simulink model "sm_planetary_gear_testrig"  (R2026a)
settings: Solver=ode45  StopTime=30  MaxStep=0.01  AbsTol=1e-4  EnableMultiTasking=on
PreLoadFcn:
  | rad_planet = 0.26;
  | rad_sun = 0.78;
  | rad_ring = 2*rad_planet+rad_sun;
  | gear_thickness = 0.5;
  | link_thickness = 0.1;
  | rad_hole = 0.05;
InitFcn:
  | sun_xcdata=Extr_Data_Gear('external',rad_sun*2,45,rad_hole);
  | planet_xcdata=Extr_Data_Gear('external',rad_planet*2,15,rad_hole);
  | ring_xcdata=Extr_Data_Gear('internal',rad_ring*2,75,rad_ring*0.05);
undefined symbols (not defined in the file or in its folder): Local, sigbuilder_block, X, Y, Z
libraries: sm_lib x22, Multibody_Parts_Lib x15, nesl_utility x7, fl_lib x3
CloseFcn:
  | try,close(h1_sm_planetary_gear_testrig),end
  | clear h1_sm_planetary_gear_testrig
  | 
  | clear simlog_sm_planetary_gear_testrig
  | clear logsout_sm_planetary_gear_testrig
Description:
  | Planetary Gear Testrig
  | 
  | Copyright 2013-2026 The MathWorks, Inc.
settings Model: Creator=smiller  LastModifiedBy=smiller
settings DataIOCC: MaxDataPoints=20000  SignalLoggingName=logsout_sm_planetary_gear_testrig
settings DebuggingCC: UnderspecifiedInitializationDetection=Classic  PregeneratedLibrarySubsystemCodeDiagnostic=none
settings HardwareCC: ProdHWDeviceType=32-bit Generic
settings SimscapeCC: SimscapeNormalizeSystem=off  SimscapeNominalValues="[{\"value\":\"1\",\"unit\":\"A\"},{\"value\":\"1\",\"unit\":\"bar\"},{\"value\":\"1\",\"unit\":\"cm^2\"},{\"value\":\"1\",\"unit\":\"cm^3/s\"},{\"value\":\"1\",\"unit\":\"kJ/kg\"},{\"value\":\"1\",\"unit\":\"kW\"},{\"value\":\"1\",\"unit\":\"l\"},{\"value\":\"1\",\"unit\":\"N\"},{\"value\":\"1\",\"unit\":\"N*m\"},{\"value\":\"1\",\"unit\":\"V\"}]"  SimscapeLogSimulationStatistics=on  SimscapeLogName=simlog_sm_planetary_gear_testrig  SimscapeLogDataHistory=20000.0
settings ConfigurationSet: Description=SimMechanics 2G
settings ExplorerConfigSet: InternalSimMechanicsExplorerSettings="<ExplorerConfiguration><canonicalview>default</canonicalview><AnimationSetting><BasePlaybackSpeed>1.0</BasePlaybackSpeed><PlaybackSpeedFactor>4.0</PlaybackSpeedFactor></AnimationSetting><TilePanel><TileInfo><Tiles Columns=\"1\" Count=\"1\" Rows=\"1\"><Column Weight=\"1\"/><Row Weight=\"1\"/><Tile Height=\"1\" Width=\"1\" X=\"0\" Y=\"0\"/></Tiles></TileInfo><SceneInfo><SceneViewer><BGColor><R>1</R><G>1</G><B>1</B></BGColor><Camera><DoPerspective>off</DoPerspective><Position><X>1.99828155084314307</X><Y>1.0003722576482561</Y><Z>4.2039432286769749</Z></Position><Center><X>0.00967718522444371843</X><Y>-0.00673071493915866625</Y><Z>0.289800264927272178</Z></Center><Up><X>-0.134695748421889611</X><Y>0.973996605340227584</Y><Z>-0.182174828510363152</Z></Up><ViewLimDist>1</ViewLimDist><YLim>2.34587518109692095</YLim><XLim>2.44514384132151186</XLim></Camera></SceneViewer></SceneInfo></TilePanel><MechEditorPanel><Cameras/><GfxPanelCameraMap/><VideoCreator><PlaybackSpeedRatio>1.0</PlaybackSpeedRatio><FrameRate>30</FrameRate><VideoFormat>Motion JPEG AVI</VideoFormat><FrameSize>auto</FrameSize></VideoCreator></MechEditorPanel></ExplorerConfiguration>"

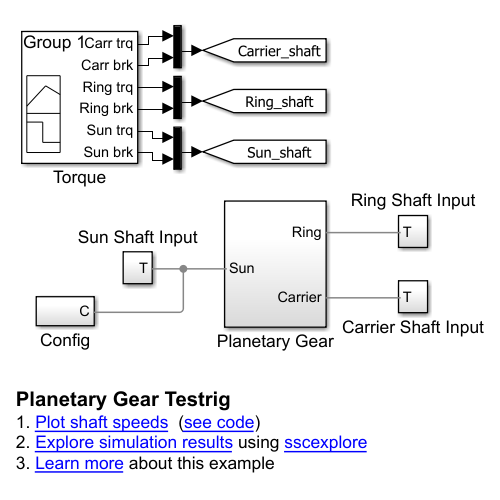
[thumbnail: Simulink's stored preview of the top-level diagram]
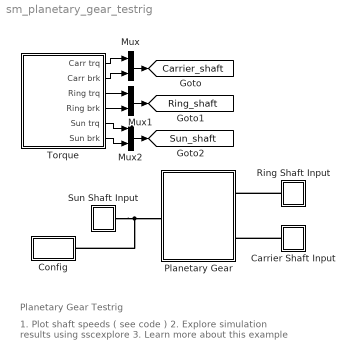
== system sm_planetary_gear_testrig ==
  note: Planetary Gear Testrig
  note: 1. Plot shaft speeds ( see code )
      | 2. Explore simulation results using sscexplore
      | 3. Learn more about this example
  Carrier Shaft Input : Subsystem
  Config : Subsystem
  Mux : Mux  Inputs=2
  Mux1 : Mux  Inputs=2
  Mux2 : Mux  Inputs=2
  Planetary Gear : Subsystem  Tag=PublishSubsystem
  Ring Shaft Input : Subsystem
  Sun Shaft Input : Subsystem  Tag=PublishSubsystem
  Torque : Subsystem  Tag=STV Subsys  LoadFcn=sigbuilder_block('load');  StartFcn=sigbuilder_block('start');  StopFcn=sigbuilder_block('stop');  ClipboardFcn=sigbuilder_block('clipboard');  mask(Sigbuilder block){tuvar=[0:10]}
      mask help: Simulink:masks:SigbuilderBlock_MD
      mask init:
      | if ~strcmp(get_param(bdroot(gcbh),'SimulationStatus'),'stopped') tuvar = sigbuilder_block('maskInit'); end
      settings: CopyFcn=sigbuilder_block('copy');  DeleteFcn=sigbuilder_block('delete');  ModelCloseFcn=sigbuilder_block('modelClose');  PreSaveFcn=sigbuilder_block('preSave');  PauseFcn=sigbuilder_block('pause');  ContinueFcn=sigbuilder_block('continue');  NameChangeFcn=sigbuilder_block('namechange');  OpenFcn=sigbuilder_block('open',[23.4 13.8 618.6 562.8 ]);  CloseFcn=sigbuilder_block('close');
      mask Display: plot(0, 0, 100, 100,[2, 2, 32, 32, 2], [68, 8, 8, 68, 68],[32, 2], [38, 38], [32, 19, 2],[53, 60, 44], [32, 17, 17, 2],[16, 16, 31, 31]);txt = getActiveGroup(gcbh);text(2, 100, txt,'verticalAlignment', 'top');
  tag scope: Carrier_shaft=global, Ring_shaft=global, Sun_shaft=global
  wires:
  Torque/1(Carr trq) -> Mux/1
  Torque/2(Carr brk) -> Mux/2
  Mux/1 -> [Carrier_shaft]
  Mux1/1 -> [Ring_shaft]
  Torque/3(Ring trq) -> Mux1/1
  Torque/4(Ring brk) -> Mux1/2
  Mux2/1 -> [Sun_shaft]
  Torque/5(Sun trq) -> Mux2/1
  Torque/6(Sun brk) -> Mux2/2
  connections:
  Sun Shaft Input/RConn1 -- Planetary Gear/LConn1 -- Config/LConn1
  Carrier Shaft Input/RConn1 -- Planetary Gear/RConn2
  Ring Shaft Input/RConn1 -- Planetary Gear/RConn1

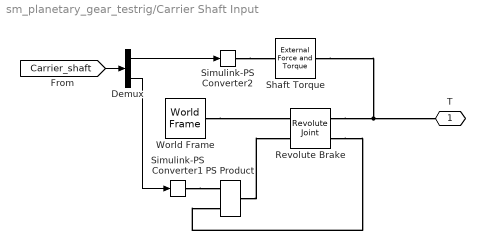
== system sm_planetary_gear_testrig/Carrier Shaft Input ==
  Demux : Demux  Outputs=2
  PS Product : fl_lib/Physical Signals/Functions/PS Product
  Revolute Brake : sm_lib/Joints/Revolute Joint  JointMode=Normal  CompositeWrenchDir=FollowerOnBase  CompositeWrenchFrame=BaseFrame  SenseConstraintForce=off  SenseConstraintTorque=off  SenseTotalForce=off  SenseTotalTorque=off  PositionTargetSpecify=off  PositionTargetPriority=High  PositionTargetValue=0  PositionTargetValueUnits=deg  VelocityTargetSpecify=off  VelocityTargetPriority=High  VelocityTargetValue=0  VelocityTargetValueUnits=deg/s  EquilibriumPosition=0  EquilibriumPositionUnits=deg  SpringStiffness=0  SpringStiffnessUnits=N*m/deg  DampingCoefficient=0  DampingCoefficientUnits=N*m/(deg/s)  LowerLimitSpecify=off  LowerLimitBound=-90  LowerLimitBoundUnits=deg  LowerLimitStiffness=1e4  LowerLimitStiffnessUnits=N*m/deg  LowerLimitDamping=10  LowerLimitDampingUnits=N*m/(deg/s)  LowerLimitTransitionRegionWidth=0.1  LowerLimitTransitionRegionWidthUnits=deg  UpperLimitSpecify=off  UpperLimitBound=90  UpperLimitBoundUnits=deg  UpperLimitStiffness=1e4  UpperLimitStiffnessUnits=N*m/deg  UpperLimitDamping=10  UpperLimitDampingUnits=N*m/(deg/s)  UpperLimitTransitionRegionWidth=0.1  UpperLimitTransitionRegionWidthUnits=deg  TorqueActuationMode=InputTorque  MotionActuationMode=ComputedMotion  SensePosition=off  SenseVelocity=on  SenseAcceleration=off  SenseTorqueForce=off  SenseLowerLimitTorqueForce=off  SenseUpperLimitTorqueForce=off
  Shaft Torque : sm_lib/Forces and Torques/External Force and Torque  EnableForceX=off  EnableForceY=off  EnableForceZ=off  EnableForce=off  ForceResolutionFrame=AttachedFrame  EnableTorqueX=off  EnableTorqueY=off  EnableTorqueZ=on  EnableTorque=off  TorqueResolutionFrame=AttachedFrame
  Simulink-PS Converter1 : nesl_utility/Simulink-PS Converter  PhysicalDomain=network_engine_domain  SubClassName=ps_input  LeftPortType=input  RightPortType=output  PseudoPeriodic=off  Frequencies=[]  NoiseDistribution=none  NoiseParameters=[]  Unit=N*m/(rad/s)  AffineConversion=off  FilteringAndDerivatives=provide  SimscapeFilterOrder=1  InputFilterTimeConstant=0.001  UdotUserProvided=0
  Simulink-PS Converter2 : nesl_utility/Simulink-PS Converter  PhysicalDomain=network_engine_domain  SubClassName=ps_input  LeftPortType=input  RightPortType=output  PseudoPeriodic=off  Frequencies=[]  NoiseDistribution=none  NoiseParameters=[]  Unit=1  AffineConversion=off  FilteringAndDerivatives=provide  SimscapeFilterOrder=1  InputFilterTimeConstant=0.001  UdotUserProvided=0
  World Frame : sm_lib/Frames and Transforms/World Frame
  T : PMIOPort  Side=Right
  wires:
  Demux/1 -> Simulink-PS Converter2/1
  Demux/2 -> Simulink-PS Converter1/1
  [Carrier_shaft] -> Demux/1
  connections:
  World Frame/RConn1 -- Revolute Brake/LConn1
  Simulink-PS Converter2/RConn1 -- Shaft Torque/LConn1
  Revolute Brake/RConn1 -- Shaft Torque/RConn1 -- T/RConn1
  Revolute Brake/RConn2 -- PS Product/LConn1
  PS Product/RConn1 -- Revolute Brake/LConn2
  Simulink-PS Converter1/RConn1 -- PS Product/LConn2

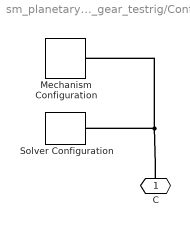
== system sm_planetary_gear_testrig/Config ==
  Mechanism Configuration : sm_lib/Utilities/Mechanism Configuration  UniformGravity=Constant  GravityVector=[0 0 0]  GravityVectorUnits=m/s^2  LinearizationDelta=0.001  JointModeTransitionNonlinearIterations=2
  Solver Configuration : nesl_utility/Solver Configuration  PhysicalDomain=network_engine_domain  SubClassName=solver  LeftPortType=input  RightPortType=generic  Tones=[]  Harmonics=[]  SimulateNoise=off  Profile=off  UseLocalSampling=off  EnableSwitchedLinearOptims=on  FrequencyDomain=off  UseCCode=off  RelTol=0.001  AbsTol=1e-06  MinStep=1e-09  ToWorkspace=off  RevertToSquareIcSolve=off  NumHomotopyIterations=100  PhasorMode=off  PhasorModeNumHarmonics=1  ConsistencySolver=NEWTON_FTOL  CanonicalOrdering=UNORDERED  OptimizeIntermediates=UNOPTIMIZED  IndexReductionMethod=DerivativeReplacement  DoDC=off  ResidualTolerance=1e-9  ConsistencyTolSource=GLOBAL  ConsistencyAbsTol=0.001  ConsistencyRelTol=0.001  ConsistencyTolFactor=0.001  UseLocalSolver=off  LocalSolverChoice=NE_BACKWARD_EULER_ADVANCER  ResolveIndetEquations=on  FunctionEvalNumThread=1  LocalSolverSampleTime=.001  DoFixedCost=off  MaxNonlinIter=3  MaxModeIter=2  ComputeImpulses=off  ImpulseIterations=2  LinearAlgebra=Sparse  LinearAlgebraNumThread=0  EquationFormulation=NE_TIME_EF  DelaysMemoryBudget=1024  AutomaticFiltering=on  FilteringTimeConstant=0.001  PartitionStorageMethod=AS_NEEDED  PartitionMemoryBudget=1024  PartitionMethod=FAST  MultibodyUseLocalSolver=off  MultibodyLocalSolverChoice=ODE1  MultibodyLocalSolverSampleTime=0.001
  C : PMIOPort  Side=Left
  connections:
  Mechanism Configuration/RConn1 -- Solver Configuration/RConn1 -- C/RConn1

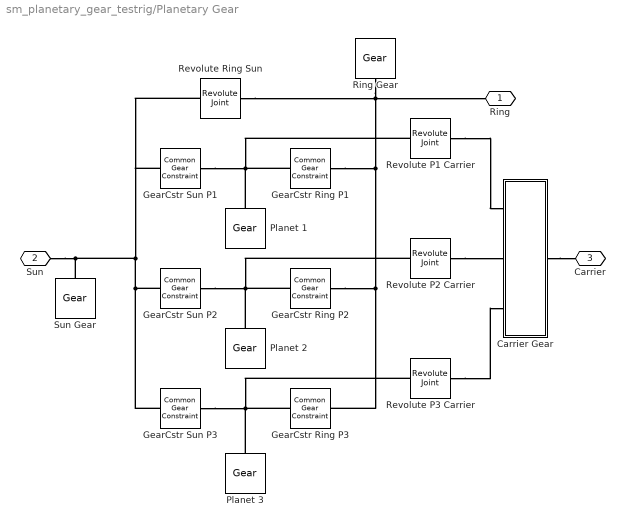
== system sm_planetary_gear_testrig/Planetary Gear ==
  Carrier Gear : Subsystem  Tag=PublishSubsystem
  GearCstr Sun P1 : sm_lib/Gears and Couplings/Gears/Common Gear Constraint  GearType=External  SpecificationType=PitchCircleRadii  CenterDistance=20.0  CenterDistanceUnits=cm  GearRatio=1.0  BaseGearRadius=rad_sun  BaseGearRadiusUnits=m  FollGearRadius=rad_planet  FollGearRadiusUnits=m  SensingForceTorqueDirection=FollowerOnBase  SensingForceTorqueResolutionFrame=BaseFrame  SenseForce=off  SenseTorque=off
  GearCstr Sun P2 : sm_lib/Gears and Couplings/Gears/Common Gear Constraint  GearType=External  SpecificationType=PitchCircleRadii  CenterDistance=20.0  CenterDistanceUnits=cm  GearRatio=1.0  BaseGearRadius=rad_sun  BaseGearRadiusUnits=m  FollGearRadius=rad_planet  FollGearRadiusUnits=m  SensingForceTorqueDirection=FollowerOnBase  SensingForceTorqueResolutionFrame=BaseFrame  SenseForce=off  SenseTorque=off
  GearCstr Sun P3 : sm_lib/Gears and Couplings/Gears/Common Gear Constraint  GearType=External  SpecificationType=PitchCircleRadii  CenterDistance=20.0  CenterDistanceUnits=cm  GearRatio=1.0  BaseGearRadius=rad_sun  BaseGearRadiusUnits=m  FollGearRadius=rad_planet  FollGearRadiusUnits=m  SensingForceTorqueDirection=FollowerOnBase  SensingForceTorqueResolutionFrame=BaseFrame  SenseForce=off  SenseTorque=off
  GearCstr Ring P1 : sm_lib/Gears and Couplings/Gears/Common Gear Constraint  GearType=Internal  SpecificationType=PitchCircleRadii  CenterDistance=20.0  CenterDistanceUnits=cm  GearRatio=1.0  BaseGearRadius=rad_ring  BaseGearRadiusUnits=m  FollGearRadius=rad_planet  FollGearRadiusUnits=m  SensingForceTorqueDirection=FollowerOnBase  SensingForceTorqueResolutionFrame=BaseFrame  SenseForce=off  SenseTorque=off
  GearCstr Ring P2 : sm_lib/Gears and Couplings/Gears/Common Gear Constraint  GearType=Internal  SpecificationType=PitchCircleRadii  CenterDistance=20.0  CenterDistanceUnits=cm  GearRatio=1.0  BaseGearRadius=rad_ring  BaseGearRadiusUnits=m  FollGearRadius=rad_planet  FollGearRadiusUnits=m  SensingForceTorqueDirection=FollowerOnBase  SensingForceTorqueResolutionFrame=BaseFrame  SenseForce=off  SenseTorque=off
  GearCstr Ring P3 : sm_lib/Gears and Couplings/Gears/Common Gear Constraint  GearType=Internal  SpecificationType=PitchCircleRadii  CenterDistance=20.0  CenterDistanceUnits=cm  GearRatio=1.0  BaseGearRadius=rad_ring  BaseGearRadiusUnits=m  FollGearRadius=rad_planet  FollGearRadiusUnits=m  SensingForceTorqueDirection=FollowerOnBase  SensingForceTorqueResolutionFrame=BaseFrame  SenseForce=off  SenseTorque=off
  Planet 1 : Multibody_Parts_Lib/Gears/Gear  popup_gear_type=External  gear_pd=rad_planet*2  gear_nt=15  gear_th=gear_thickness  gear_rh=rad_hole  gear_rt=0.02  gear_rho=7000  gear_clr=[0.8 0.8 0.8]  gear_opc=1  popup_ad_dd=Default  gear_ad=0.125/12  gear_dd=1.157*0.125/12  popup_markings=Two  mark_radius_range=[0.6 0.7]  mark_angle_range=60  mark_color=[1 1 1]*0.2
      settings: SourceProductName=Simscape Multibody Parts Library
  Planet 2 : Multibody_Parts_Lib/Gears/Gear  popup_gear_type=External  gear_pd=rad_planet*2  gear_nt=15  gear_th=gear_thickness  gear_rh=rad_hole  gear_rt=0.02  gear_rho=7000  gear_clr=[0.8 0.8 0.8]  gear_opc=1  popup_ad_dd=Default  gear_ad=0.125/12  gear_dd=1.157*0.125/12  popup_markings=Two  mark_radius_range=[0.6 0.7]  mark_angle_range=60  mark_color=[1 1 1]*0.2
      settings: SourceProductName=Simscape Multibody Parts Library
  Planet 3 : Multibody_Parts_Lib/Gears/Gear  popup_gear_type=External  gear_pd=rad_planet*2  gear_nt=15  gear_th=gear_thickness  gear_rh=rad_hole  gear_rt=0.02  gear_rho=7000  gear_clr=[0.8 0.8 0.8]  gear_opc=1  popup_ad_dd=Default  gear_ad=0.125/12  gear_dd=1.157*0.125/12  popup_markings=Two  mark_radius_range=[0.6 0.7]  mark_angle_range=60  mark_color=[1 1 1]*0.2
      settings: SourceProductName=Simscape Multibody Parts Library
  Revolute P1 Carrier : sm_lib/Joints/Revolute Joint  JointMode=Normal  CompositeWrenchDir=FollowerOnBase  CompositeWrenchFrame=BaseFrame  SenseConstraintForce=off  SenseConstraintTorque=off  SenseTotalForce=off  SenseTotalTorque=off  PositionTargetSpecify=off  PositionTargetPriority=High  PositionTargetValue=0  PositionTargetValueUnits=deg  VelocityTargetSpecify=off  VelocityTargetPriority=High  VelocityTargetValue=0  VelocityTargetValueUnits=deg/s  EquilibriumPosition=0  EquilibriumPositionUnits=deg  SpringStiffness=0  SpringStiffnessUnits=N*m/deg  DampingCoefficient=0  DampingCoefficientUnits=N*m/(deg/s)  LowerLimitSpecify=off  LowerLimitBound=-90  LowerLimitBoundUnits=deg  LowerLimitStiffness=1e4  LowerLimitStiffnessUnits=N*m/deg  LowerLimitDamping=10  LowerLimitDampingUnits=N*m/(deg/s)  LowerLimitTransitionRegionWidth=0.1  LowerLimitTransitionRegionWidthUnits=deg  UpperLimitSpecify=off  UpperLimitBound=90  UpperLimitBoundUnits=deg  UpperLimitStiffness=1e4  UpperLimitStiffnessUnits=N*m/deg  UpperLimitDamping=10  UpperLimitDampingUnits=N*m/(deg/s)  UpperLimitTransitionRegionWidth=0.1  UpperLimitTransitionRegionWidthUnits=deg  TorqueActuationMode=NoTorque  MotionActuationMode=ComputedMotion  SensePosition=off  SenseVelocity=off  SenseAcceleration=off  SenseTorqueForce=off  SenseLowerLimitTorqueForce=off  SenseUpperLimitTorqueForce=off
  Revolute P2 Carrier : sm_lib/Joints/Revolute Joint  JointMode=Normal  CompositeWrenchDir=FollowerOnBase  CompositeWrenchFrame=BaseFrame  SenseConstraintForce=off  SenseConstraintTorque=off  SenseTotalForce=off  SenseTotalTorque=off  PositionTargetSpecify=off  PositionTargetPriority=High  PositionTargetValue=0  PositionTargetValueUnits=deg  VelocityTargetSpecify=off  VelocityTargetPriority=High  VelocityTargetValue=0  VelocityTargetValueUnits=deg/s  EquilibriumPosition=0  EquilibriumPositionUnits=deg  SpringStiffness=0  SpringStiffnessUnits=N*m/deg  DampingCoefficient=0  DampingCoefficientUnits=N*m/(deg/s)  LowerLimitSpecify=off  LowerLimitBound=-90  LowerLimitBoundUnits=deg  LowerLimitStiffness=1e4  LowerLimitStiffnessUnits=N*m/deg  LowerLimitDamping=10  LowerLimitDampingUnits=N*m/(deg/s)  LowerLimitTransitionRegionWidth=0.1  LowerLimitTransitionRegionWidthUnits=deg  UpperLimitSpecify=off  UpperLimitBound=90  UpperLimitBoundUnits=deg  UpperLimitStiffness=1e4  UpperLimitStiffnessUnits=N*m/deg  UpperLimitDamping=10  UpperLimitDampingUnits=N*m/(deg/s)  UpperLimitTransitionRegionWidth=0.1  UpperLimitTransitionRegionWidthUnits=deg  TorqueActuationMode=NoTorque  MotionActuationMode=ComputedMotion  SensePosition=off  SenseVelocity=off  SenseAcceleration=off  SenseTorqueForce=off  SenseLowerLimitTorqueForce=off  SenseUpperLimitTorqueForce=off
  Revolute P3 Carrier : sm_lib/Joints/Revolute Joint  JointMode=Normal  CompositeWrenchDir=FollowerOnBase  CompositeWrenchFrame=BaseFrame  SenseConstraintForce=off  SenseConstraintTorque=off  SenseTotalForce=off  SenseTotalTorque=off  PositionTargetSpecify=off  PositionTargetPriority=High  PositionTargetValue=0  PositionTargetValueUnits=deg  VelocityTargetSpecify=off  VelocityTargetPriority=High  VelocityTargetValue=0  VelocityTargetValueUnits=deg/s  EquilibriumPosition=0  EquilibriumPositionUnits=deg  SpringStiffness=0  SpringStiffnessUnits=N*m/deg  DampingCoefficient=0  DampingCoefficientUnits=N*m/(deg/s)  LowerLimitSpecify=off  LowerLimitBound=-90  LowerLimitBoundUnits=deg  LowerLimitStiffness=1e4  LowerLimitStiffnessUnits=N*m/deg  LowerLimitDamping=10  LowerLimitDampingUnits=N*m/(deg/s)  LowerLimitTransitionRegionWidth=0.1  LowerLimitTransitionRegionWidthUnits=deg  UpperLimitSpecify=off  UpperLimitBound=90  UpperLimitBoundUnits=deg  UpperLimitStiffness=1e4  UpperLimitStiffnessUnits=N*m/deg  UpperLimitDamping=10  UpperLimitDampingUnits=N*m/(deg/s)  UpperLimitTransitionRegionWidth=0.1  UpperLimitTransitionRegionWidthUnits=deg  TorqueActuationMode=NoTorque  MotionActuationMode=ComputedMotion  SensePosition=off  SenseVelocity=off  SenseAcceleration=off  SenseTorqueForce=off  SenseLowerLimitTorqueForce=off  SenseUpperLimitTorqueForce=off
  Revolute Ring Sun : sm_lib/Joints/Revolute Joint  JointMode=Normal  CompositeWrenchDir=FollowerOnBase  CompositeWrenchFrame=BaseFrame  SenseConstraintForce=off  SenseConstraintTorque=off  SenseTotalForce=off  SenseTotalTorque=off  PositionTargetSpecify=on  PositionTargetPriority=High  PositionTargetValue=0  PositionTargetValueUnits=deg  VelocityTargetSpecify=off  VelocityTargetPriority=High  VelocityTargetValue=0  VelocityTargetValueUnits=deg/s  EquilibriumPosition=0  EquilibriumPositionUnits=deg  SpringStiffness=0  SpringStiffnessUnits=N*m/deg  DampingCoefficient=0  DampingCoefficientUnits=N*m/(deg/s)  LowerLimitSpecify=off  LowerLimitBound=-90  LowerLimitBoundUnits=deg  LowerLimitStiffness=1e4  LowerLimitStiffnessUnits=N*m/deg  LowerLimitDamping=10  LowerLimitDampingUnits=N*m/(deg/s)  LowerLimitTransitionRegionWidth=0.1  LowerLimitTransitionRegionWidthUnits=deg  UpperLimitSpecify=off  UpperLimitBound=90  UpperLimitBoundUnits=deg  UpperLimitStiffness=1e4  UpperLimitStiffnessUnits=N*m/deg  UpperLimitDamping=10  UpperLimitDampingUnits=N*m/(deg/s)  UpperLimitTransitionRegionWidth=0.1  UpperLimitTransitionRegionWidthUnits=deg  TorqueActuationMode=NoTorque  MotionActuationMode=ComputedMotion  SensePosition=off  SenseVelocity=off  SenseAcceleration=off  SenseTorqueForce=off  SenseLowerLimitTorqueForce=off  SenseUpperLimitTorqueForce=off
  Ring Gear : Multibody_Parts_Lib/Gears/Gear  popup_gear_type=Internal  gear_pd=rad_ring*2  gear_nt=75  gear_th=gear_thickness  gear_rh=0.05  gear_rt=rad_ring*0.1  gear_rho=7000  gear_clr=[0.0 0.4 0.6]  gear_opc=1  popup_ad_dd=Default  gear_ad=0.125/12  gear_dd=1.157*0.125/12  popup_markings=Two  mark_radius_range=[1.06 1.1]  mark_angle_range=60  mark_color=[1 1 1]
      settings: SourceProductName=Simscape Multibody Parts Library
  Sun Gear : Multibody_Parts_Lib/Gears/Gear  popup_gear_type=External  gear_pd=rad_sun*2  gear_nt=45  gear_th=gear_thickness  gear_rh=rad_hole  gear_rt=0.02  gear_rho=7000  gear_clr=[0.8 0.8 0.3]  gear_opc=1  popup_ad_dd=Default  gear_ad=0.125/12  gear_dd=1.157*0.125/12  popup_markings=Two  mark_radius_range=[0.6 0.7]  mark_angle_range=60  mark_color=[1 1 1]*0.2
      settings: SourceProductName=Simscape Multibody Parts Library
  Ring : PMIOPort  Side=Right
  Sun : PMIOPort  Port=2  Side=Left
  Carrier : PMIOPort  Port=3  Side=Right
  connections:
  Carrier Gear/RConn1 -- Carrier/RConn1
  GearCstr Ring P2/RConn1 -- Revolute P2 Carrier/LConn1 -- Planet 2/RConn1 -- GearCstr Sun P2/RConn1
  GearCstr Ring P1/RConn1 -- Revolute P1 Carrier/LConn1 -- Planet 1/RConn1 -- GearCstr Sun P1/RConn1
  GearCstr Ring P3/RConn1 -- Revolute P3 Carrier/LConn1 -- Planet 3/RConn1 -- GearCstr Sun P3/RConn1
  GearCstr Sun P2/LConn1 -- GearCstr Sun P3/LConn1 -- GearCstr Sun P1/LConn1 -- Revolute Ring Sun/RConn1 -- Sun/RConn1 -- Sun Gear/RConn1
  Revolute Ring Sun/LConn1 -- Ring/RConn1 -- Ring Gear/RConn1 -- GearCstr Ring P1/LConn1 -- GearCstr Ring P3/LConn1 -- GearCstr Ring P2/LConn1
  Revolute P1 Carrier/RConn1 -- Carrier Gear/LConn1
  Revolute P2 Carrier/RConn1 -- Carrier Gear/LConn2
  Revolute P3 Carrier/RConn1 -- Carrier Gear/LConn3

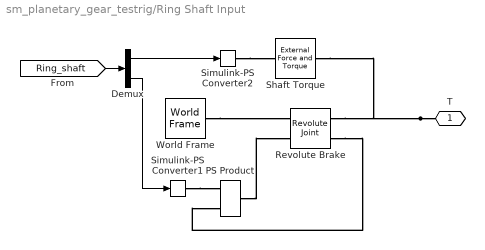
== system sm_planetary_gear_testrig/Ring Shaft Input ==
  Demux : Demux  Outputs=2
  PS Product : fl_lib/Physical Signals/Functions/PS Product
  Revolute Brake : sm_lib/Joints/Revolute Joint  JointMode=Normal  CompositeWrenchDir=FollowerOnBase  CompositeWrenchFrame=BaseFrame  SenseConstraintForce=off  SenseConstraintTorque=off  SenseTotalForce=off  SenseTotalTorque=off  PositionTargetSpecify=off  PositionTargetPriority=High  PositionTargetValue=0  PositionTargetValueUnits=deg  VelocityTargetSpecify=off  VelocityTargetPriority=High  VelocityTargetValue=0  VelocityTargetValueUnits=deg/s  EquilibriumPosition=0  EquilibriumPositionUnits=deg  SpringStiffness=0  SpringStiffnessUnits=N*m/deg  DampingCoefficient=0  DampingCoefficientUnits=N*m/(deg/s)  LowerLimitSpecify=off  LowerLimitBound=-90  LowerLimitBoundUnits=deg  LowerLimitStiffness=1e4  LowerLimitStiffnessUnits=N*m/deg  LowerLimitDamping=10  LowerLimitDampingUnits=N*m/(deg/s)  LowerLimitTransitionRegionWidth=0.1  LowerLimitTransitionRegionWidthUnits=deg  UpperLimitSpecify=off  UpperLimitBound=90  UpperLimitBoundUnits=deg  UpperLimitStiffness=1e4  UpperLimitStiffnessUnits=N*m/deg  UpperLimitDamping=10  UpperLimitDampingUnits=N*m/(deg/s)  UpperLimitTransitionRegionWidth=0.1  UpperLimitTransitionRegionWidthUnits=deg  TorqueActuationMode=InputTorque  MotionActuationMode=ComputedMotion  SensePosition=off  SenseVelocity=on  SenseAcceleration=off  SenseTorqueForce=off  SenseLowerLimitTorqueForce=off  SenseUpperLimitTorqueForce=off
  Shaft Torque : sm_lib/Forces and Torques/External Force and Torque  EnableForceX=off  EnableForceY=off  EnableForceZ=off  EnableForce=off  ForceResolutionFrame=AttachedFrame  EnableTorqueX=off  EnableTorqueY=off  EnableTorqueZ=on  EnableTorque=off  TorqueResolutionFrame=AttachedFrame
  Simulink-PS Converter1 : nesl_utility/Simulink-PS Converter  PhysicalDomain=network_engine_domain  SubClassName=ps_input  LeftPortType=input  RightPortType=output  PseudoPeriodic=off  Frequencies=[]  NoiseDistribution=none  NoiseParameters=[]  Unit=N*m/(rad/s)  AffineConversion=off  FilteringAndDerivatives=provide  SimscapeFilterOrder=1  InputFilterTimeConstant=0.001  UdotUserProvided=0
  Simulink-PS Converter2 : nesl_utility/Simulink-PS Converter  PhysicalDomain=network_engine_domain  SubClassName=ps_input  LeftPortType=input  RightPortType=output  PseudoPeriodic=off  Frequencies=[]  NoiseDistribution=none  NoiseParameters=[]  Unit=1  AffineConversion=off  FilteringAndDerivatives=provide  SimscapeFilterOrder=1  InputFilterTimeConstant=0.001  UdotUserProvided=0
  World Frame : sm_lib/Frames and Transforms/World Frame
  T : PMIOPort  Side=Right
  wires:
  [Ring_shaft] -> Demux/1
  Demux/2 -> Simulink-PS Converter1/1
  Demux/1 -> Simulink-PS Converter2/1
  connections:
  Simulink-PS Converter1/RConn1 -- PS Product/LConn2
  PS Product/RConn1 -- Revolute Brake/LConn2
  Revolute Brake/RConn2 -- PS Product/LConn1
  T/RConn1 -- Shaft Torque/RConn1 -- Revolute Brake/RConn1
  Simulink-PS Converter2/RConn1 -- Shaft Torque/LConn1
  World Frame/RConn1 -- Revolute Brake/LConn1

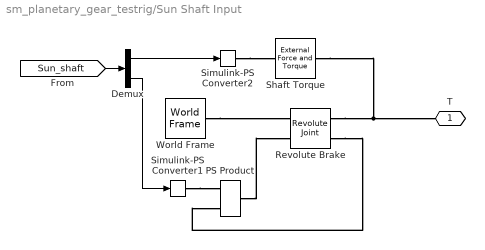
== system sm_planetary_gear_testrig/Sun Shaft Input ==
  Demux : Demux  Outputs=2
  PS Product : fl_lib/Physical Signals/Functions/PS Product
  Revolute Brake : sm_lib/Joints/Revolute Joint  JointMode=Normal  CompositeWrenchDir=FollowerOnBase  CompositeWrenchFrame=BaseFrame  SenseConstraintForce=off  SenseConstraintTorque=off  SenseTotalForce=off  SenseTotalTorque=off  PositionTargetSpecify=off  PositionTargetPriority=High  PositionTargetValue=0  PositionTargetValueUnits=deg  VelocityTargetSpecify=off  VelocityTargetPriority=High  VelocityTargetValue=0  VelocityTargetValueUnits=deg/s  EquilibriumPosition=0  EquilibriumPositionUnits=deg  SpringStiffness=0  SpringStiffnessUnits=N*m/deg  DampingCoefficient=0  DampingCoefficientUnits=N*m/(deg/s)  LowerLimitSpecify=off  LowerLimitBound=-90  LowerLimitBoundUnits=deg  LowerLimitStiffness=1e4  LowerLimitStiffnessUnits=N*m/deg  LowerLimitDamping=10  LowerLimitDampingUnits=N*m/(deg/s)  LowerLimitTransitionRegionWidth=0.1  LowerLimitTransitionRegionWidthUnits=deg  UpperLimitSpecify=off  UpperLimitBound=90  UpperLimitBoundUnits=deg  UpperLimitStiffness=1e4  UpperLimitStiffnessUnits=N*m/deg  UpperLimitDamping=10  UpperLimitDampingUnits=N*m/(deg/s)  UpperLimitTransitionRegionWidth=0.1  UpperLimitTransitionRegionWidthUnits=deg  TorqueActuationMode=InputTorque  MotionActuationMode=ComputedMotion  SensePosition=off  SenseVelocity=on  SenseAcceleration=off  SenseTorqueForce=off  SenseLowerLimitTorqueForce=off  SenseUpperLimitTorqueForce=off
  Shaft Torque : sm_lib/Forces and Torques/External Force and Torque  EnableForceX=off  EnableForceY=off  EnableForceZ=off  EnableForce=off  ForceResolutionFrame=AttachedFrame  EnableTorqueX=off  EnableTorqueY=off  EnableTorqueZ=on  EnableTorque=off  TorqueResolutionFrame=AttachedFrame
  Simulink-PS Converter1 : nesl_utility/Simulink-PS Converter  PhysicalDomain=network_engine_domain  SubClassName=ps_input  LeftPortType=input  RightPortType=output  PseudoPeriodic=off  Frequencies=[]  NoiseDistribution=none  NoiseParameters=[]  Unit=N*m/(rad/s)  AffineConversion=off  FilteringAndDerivatives=provide  SimscapeFilterOrder=1  InputFilterTimeConstant=0.001  UdotUserProvided=0
  Simulink-PS Converter2 : nesl_utility/Simulink-PS Converter  PhysicalDomain=network_engine_domain  SubClassName=ps_input  LeftPortType=input  RightPortType=output  PseudoPeriodic=off  Frequencies=[]  NoiseDistribution=none  NoiseParameters=[]  Unit=1  AffineConversion=off  FilteringAndDerivatives=provide  SimscapeFilterOrder=1  InputFilterTimeConstant=0.001  UdotUserProvided=0
  World Frame : sm_lib/Frames and Transforms/World Frame
  T : PMIOPort  Side=Right
  wires:
  Demux/1 -> Simulink-PS Converter2/1
  Demux/2 -> Simulink-PS Converter1/1
  [Sun_shaft] -> Demux/1
  connections:
  World Frame/RConn1 -- Revolute Brake/LConn1
  Simulink-PS Converter2/RConn1 -- Shaft Torque/LConn1
  Revolute Brake/RConn1 -- Shaft Torque/RConn1 -- T/RConn1
  Revolute Brake/RConn2 -- PS Product/LConn1
  PS Product/RConn1 -- Revolute Brake/LConn2
  Simulink-PS Converter1/RConn1 -- PS Product/LConn2

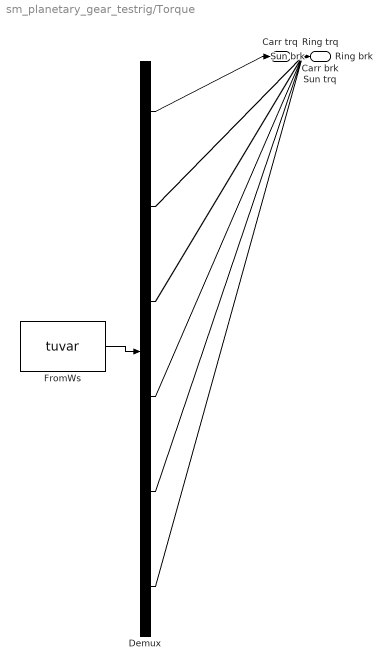
== system sm_planetary_gear_testrig/Torque ==
  Demux : Demux  Tag=STV Demux  Outputs=6
      settings: DisplayOption=none
  FromWs : FromWorkspace  Tag=STV FromWs  VariableName=tuvar
      SigBuilderData=|
      | common.afterFinalStr = 'Extrapolate'
      | common.sampleTime = 0
      | dataSet.timeRange = [0 30]
      | dataSet.name = 'Group 1'
      | sbobj.Groups.Name = 'Group 1'
      | sbobj.Groups.Signals(1).Name = 'Carr trq'
      | sbobj.Groups.Signals(1).XData = [0 1 3 4 6 11 11 13 13 16 16 18 18 30]
      | sbobj.Groups.Signals(1).YData = [0 0 0 0 0 0 -3000 -3000 0 0 -3000 -3000 0 0]
      | sbobj.Groups.Signals(2).Name = 'Carr brk'
      | sbobj.Groups.Signals(2).XData = [0 0.5 0.5 5 5 9 9 10 10 14 14 15 15 19 19 20 20 24 24 25 25 25.5 25.5 30]
      | sbobj.Groups.Signals(2).YData = [0 0 -1000000 -1000000 0 0 -1000000 -1000000 0 0 -1000000 -1000000 0 0 -1000000 -1000000 0 0 -1000000 -1000000 0 0 -1000000 -1000000]
      | sbobj.Groups.Signals(3).Name = 'Ring trq'
      | sbobj.Groups.Signals(3).XData = [0 21 21 23 23 26 26 28 28 30]
      | sbobj.Groups.Signals(3).YData = [0 0 2000 2000 0 0 2000 2000 0 0]
      | sbobj.Groups.Signals(4).Name = 'Ring brk'
      | sbobj.Groups.Signals(4).XData = [0 4 4 5 5 5.5 5.5 10 10 14 14 15 15 15.5 15.5 20 20 24 24 25 25 29 29 30]
      | sbobj.Groups.Signals(4).YData = [0 0 -1000000 -1000000 0 0 -1000000 -1000000 0 0 -1000000 -1000000 0 0 -1000000 -1000000 0 0 -1000000 -1000000 0 0 -1000000 -1000000]
      | sbobj.Groups.Signals(5).Name = 'Sun trq'
      | sbobj.Groups.Signals(5).XData = [0 1 1 3 3 6 6 8 8 30]
      | sbobj.Groups.Signals(5).YData = [0 0 1000 1000 0 0 1000 1000 0 0]
      | sbobj.Groups.Signals(6).Name = 'Sun brk'
      | sbobj.Groups.Signals(6).XData = [0 4 4 5 5 9 9 10 10 10.5 10.5 15 15 19 19 20 20 20.5 20.5 25 25 29 29 30]
      | sbobj.Groups.Signals(6).YData = [0 0 -100000 -100000 1 1 -100000 -100000 1 1 -100000 -100000 1 1 -100000 -100000 1 1 -100000 -100000 1 1 -100000 -100000]
      | sbobj.Groups.TimeRange = [0 30]
  Carr trq : Outport  Tag=STV Outport  VectorParamsAs1DForOutWhenUnconnected=off
  Carr brk : Outport  Tag=STV Outport  Port=2  VectorParamsAs1DForOutWhenUnconnected=off
  Ring trq : Outport  Tag=STV Outport  Port=3  VectorParamsAs1DForOutWhenUnconnected=off
  Ring brk : Outport  Tag=STV Outport  Port=4  VectorParamsAs1DForOutWhenUnconnected=off
  Sun trq : Outport  Tag=STV Outport  Port=5  VectorParamsAs1DForOutWhenUnconnected=off
  Sun brk : Outport  Tag=STV Outport  Port=6  VectorParamsAs1DForOutWhenUnconnected=off
  wires:
  FromWs/1 -> Demux/1
  Demux/1 -> Carr trq/1
  Demux/2 -> Carr brk/1
  Demux/3 -> Ring trq/1
  Demux/4 -> Ring brk/1
  Demux/5 -> Sun trq/1
  Demux/6 -> Sun brk/1

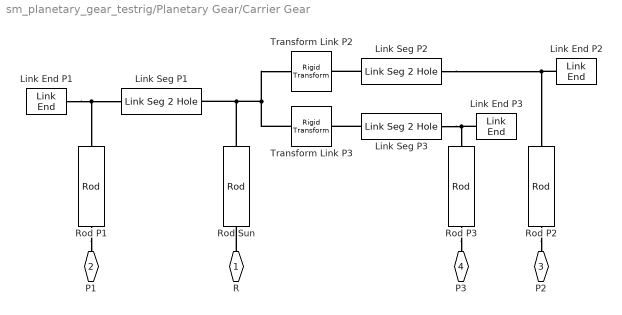
== system sm_planetary_gear_testrig/Planetary Gear/Carrier Gear ==
  Link End P1 : Multibody_Parts_Lib/Linkages/Link End  circ_radout=rad_hole*2  circ_radin=rad_hole  popup_holelr=+X  deg_1=-90  deg_2=90  circ_len=link_thickness  circ_rho=7000  circ_color=[0.5 0.5 0.5]  circ_opc=1
      settings: SourceProductName=Simscape Multibody Parts Library
  Link End P2 : Multibody_Parts_Lib/Linkages/Link End  circ_radout=rad_hole*2  circ_radin=rad_hole  popup_holelr=+X  deg_1=-90  deg_2=90  circ_len=link_thickness  circ_rho=7000  circ_color=[0.5 0.5 0.5]  circ_opc=1
      settings: SourceProductName=Simscape Multibody Parts Library
  Link End P3 : Multibody_Parts_Lib/Linkages/Link End  circ_radout=rad_hole*2  circ_radin=rad_hole  popup_holelr=+X  deg_1=-90  deg_2=90  circ_len=link_thickness  circ_rho=7000  circ_color=[0.5 0.5 0.5]  circ_opc=1
      settings: SourceProductName=Simscape Multibody Parts Library
  Link Seg P1 : Multibody_Parts_Lib/Linkages/Link Seg 2 Hole  link_len=rad_sun+rad_planet  link_width=rad_hole*2*2  link_radh=rad_hole  link_thickness=link_thickness  link_rho=7000  link_color=[0.5 0.5 0.5]  link_opc=1
      settings: SourceProductName=Simscape Multibody Parts Library
  Link Seg P2 : Multibody_Parts_Lib/Linkages/Link Seg 2 Hole  link_len=rad_sun+rad_planet  link_width=rad_hole*2*2  link_radh=rad_hole  link_thickness=link_thickness  link_rho=7000  link_color=[0.5 0.5 0.5]  link_opc=1
      settings: SourceProductName=Simscape Multibody Parts Library
  Link Seg P3 : Multibody_Parts_Lib/Linkages/Link Seg 2 Hole  link_len=rad_sun+rad_planet  link_width=rad_hole*2*2  link_radh=rad_hole  link_thickness=link_thickness  link_rho=7000  link_color=[0.5 0.5 0.5]  link_opc=1
      settings: SourceProductName=Simscape Multibody Parts Library
  Rod P1 : Multibody_Parts_Lib/Basic/Rod  rod_rad=rad_hole  rod_len=gear_thickness  rod_rho=7000  rod_color=[0.5 0.5 0.5]  rod_opc=1  popup_zori=Local +Z  popup_markings=None  mark_radius_range=[0.5 1.01]  mark_length_range=1.005  mark_angle_range=30  mark_color=[1 1 1]
      settings: SourceProductName=Simscape Multibody Parts Library
  Rod P2 : Multibody_Parts_Lib/Basic/Rod  rod_rad=rad_hole  rod_len=gear_thickness  rod_rho=7000  rod_color=[0.5 0.5 0.5]  rod_opc=1  popup_zori=Local +Z  popup_markings=None  mark_radius_range=[0.5 1.01]  mark_length_range=1.005  mark_angle_range=30  mark_color=[1 1 1]
      settings: SourceProductName=Simscape Multibody Parts Library
  Rod P3 : Multibody_Parts_Lib/Basic/Rod  rod_rad=rad_hole  rod_len=gear_thickness  rod_rho=7000  rod_color=[0.5 0.5 0.5]  rod_opc=1  popup_zori=Local +Z  popup_markings=None  mark_radius_range=[0.5 1.01]  mark_length_range=1.005  mark_angle_range=30  mark_color=[1 1 1]
      settings: SourceProductName=Simscape Multibody Parts Library
  Rod Sun : Multibody_Parts_Lib/Basic/Rod  rod_rad=rad_hole  rod_len=gear_thickness  rod_rho=7000  rod_color=[0.5 0.5 0.5]  rod_opc=1  popup_zori=Local +Z  popup_markings=None  mark_radius_range=[0.5 1.01]  mark_length_range=1.005  mark_angle_range=30  mark_color=[1 1 1]
      settings: SourceProductName=Simscape Multibody Parts Library
  Transform Link P2 : sm_lib/Frames and Transforms/Rigid Transform  RotationMethod=StandardAxis  FollAlignAxisA=+X  BaseAlignAxisA=+Y  FollAlignAxisB=+Y  BaseAlignAxisB=+Z  RotationStandardAxis=+Z  RotationAngle=120  RotationAngleUnits=deg  RotationArbitraryAxis=[0 0 1]  RotationSequenceAxes=FollowerAxes  RotationSequence=XYX  RotationSequenceAngles=[0 0 0]  RotationSequenceAnglesUnits=deg  RotationMatrix=[1 0 0; 0 1 0; 0 0 1]  Quaternion=[1 0 0 0]  TranslationMethod=None  TranslationCartesianOffset=[0 0 0]  TranslationCartesianOffsetUnits=m  TranslationStandardAxis=+Z  TranslationStandardOffset=0  TranslationStandardOffsetUnits=m  TranslationROffset=0  TranslationROffsetUnits=m  TranslationThetaOffset=0  TranslationThetaOffsetUnits=deg  TranslationZOffset=0  TranslationZOffsetUnits=m
  Transform Link P3 : sm_lib/Frames and Transforms/Rigid Transform  RotationMethod=StandardAxis  FollAlignAxisA=+X  BaseAlignAxisA=+Y  FollAlignAxisB=+Y  BaseAlignAxisB=+Z  RotationStandardAxis=+Z  RotationAngle=-120  RotationAngleUnits=deg  RotationArbitraryAxis=[0 0 1]  RotationSequenceAxes=FollowerAxes  RotationSequence=XYX  RotationSequenceAngles=[0 0 0]  RotationSequenceAnglesUnits=deg  RotationMatrix=[1 0 0; 0 1 0; 0 0 1]  Quaternion=[1 0 0 0]  TranslationMethod=None  TranslationCartesianOffset=[0 0 0]  TranslationCartesianOffsetUnits=m  TranslationStandardAxis=+Z  TranslationStandardOffset=0  TranslationStandardOffsetUnits=m  TranslationROffset=0  TranslationROffsetUnits=m  TranslationThetaOffset=0  TranslationThetaOffsetUnits=deg  TranslationZOffset=0  TranslationZOffsetUnits=m
  R : PMIOPort  Side=Right
  P1 : PMIOPort  Port=2  Side=Left
  P2 : PMIOPort  Port=3  Side=Left
  P3 : PMIOPort  Port=4  Side=Left
  connections:
  Rod P1/LConn1 -- P1/RConn1
  Link End P1/LConn1 -- Rod P1/RConn1 -- Link Seg P1/RConn1
  Rod Sun/RConn1 -- Transform Link P2/LConn1 -- Transform Link P3/LConn1 -- Link Seg P1/LConn1
  Link Seg P2/RConn1 -- Link End P2/LConn1 -- Rod P2/RConn1
  Link Seg P2/LConn1 -- Transform Link P2/RConn1
  R/RConn1 -- Rod Sun/LConn1
  Link Seg P3/RConn1 -- Rod P3/RConn1 -- Link End P3/LConn1
  Link Seg P3/LConn1 -- Transform Link P3/RConn1
  Rod P2/LConn1 -- P2/RConn1
  Rod P3/LConn1 -- P3/RConn1
